simulink model "quad_new_leg_raibert_strategy_v2"  (R2022b)
settings: Solver=ode15s  StartTime=0.0  StopTime=400  RelTol=1e-3
InitFcn:
  | init_quad_new_leg_raibert_strategy_v2
values from neighbouring files (symbols this model uses):
  body = 'obstacle'+string(i)    [GUIWithNavigation.m]    (also in RunModel.m)
  floorl = 20    [EnvironmentData.mat]    (also in GUIWithNavigation.m; Practice data.mat; RunModel.m)
  floorw = 20    [EnvironmentData.mat]    (also in GUIWithNavigation.m; Practice data.mat; RunModel.m)
  planner = plannerRRTStar(ss,stateValidator)    [GUIWithNavigation.m]    (also in RunModel.m)
  startx = 3    [EnvironmentData.mat]    (also in Practice data.mat = 2)
  starty = 3    [EnvironmentData.mat]    (also in Practice data.mat = 2)
  tar1Len = 10    [EnvironmentData.mat]    (also in GUIWithNavigation.m = length(target1); Practice data.mat = 13; RunModel.m = length(target1))
  target = [3 4.99844642156 6.95141646815 8.78790598722 9.67257563911 9.70990834754 10.5092252376 9.30187214417 9.05327436398 9.4 9.4 10.8486938703 ... (44 elements, 22x2)]    [EnvironmentData.mat]    (also in GUIWithNavigation.m = cat(1,target1,target2); Practice data.mat = [2 3.44057581018 5.07942513831 5.42542290116 7.21306818311 8; RunModel.m = cat(1,target1,target2))
undefined symbols (not defined in the file or in its folder): closeFingers, ctrl, Extr_Data_LinkEndHole, grabObjectAngles, grabObjectAngles2, ground, holdFingers, l1, l2, m1, m2, openFingers, readyAngles, X, Y, Z
libraries: sm_lib x277, nesl_utility x98, slpidlib x31, simulink x5, Contact_Forces_Lib x4, Parts_Lib x4, sharedtransform x2
(part 1 of 11)
settings Model: Creator=biorobotics  LastModifiedBy=Harry
settings SolverCC: AlgebraicLoopSolver=TrustRegion
settings DataIOCC: ReturnWorkspaceOutputs=off
settings DebuggingCC: UnconnectedInputMsg=warning  UnconnectedOutputMsg=warning  UnconnectedLineMsg=warning  SFMachineParentedDataDiag=warning  ArithmeticOperatorsInVariantConditions=warning
settings ModelReferenceCC: EnableRefExpFcnMdlSchedulingChecks=on
settings SFSimCC: SimUseLocalCustomCode=off  CustomCodeUndefinedFunction=UseInterfaceOnly
settings RTWCC: RTWUseLocalCustomCode=off
settings DiagnosticsConfigSet: SimMechanicsRigidlyBoundBlock=none

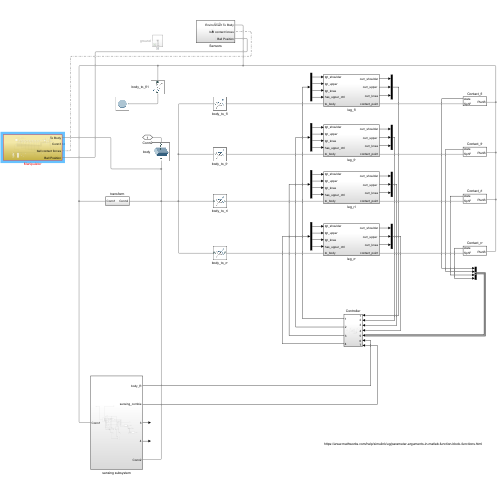
[thumbnail: Simulink's stored preview of the top-level diagram]
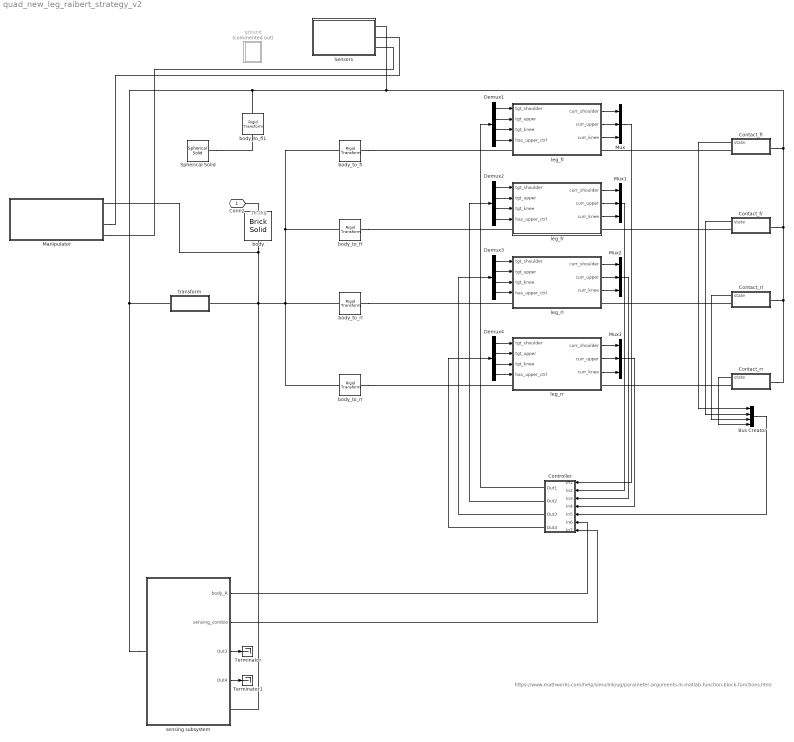
== system quad_new_leg_raibert_strategy_v2 ==
  note: 16.2kg
  note: https://www.mathworks.com/help/simulink/ug/parameter-arguments-in-matlab-function-block-functions.html
  Bus Creator : BusCreator  Inputs=4
  Contact_fl : Subsystem
  Contact_fr : Subsystem
  Contact_rl : Subsystem
  Contact_rr : Subsystem
  Controller : Subsystem
  Demux{1..4} (4 alike) : Demux
  Manipulator : Subsystem
  Mux{,1..3} (4 alike) : Mux  Inputs=3
  Sensors : Subsystem
  Spherical Solid : sm_lib/Body Elements/Spherical Solid  GraphicAmbientColor=[0.15 0.15 0.15 1.0]  BasedOnType=Density  CenterOfMass=[0 0 0]  CenterOfMassUnits=m  GraphicDiffuseColor=[0.4 0.2 0.0]  Density=1000  DensityUnits=kg/m^3  DoExposeReferenceFrame=on  GraphicEmissiveColor=[0.0 0.0 0.0 1.0]  ExportEntireGeometry=off  SerializedExposedGeometries=<ExposedGeometries/>  SerializedFrames=<Frames/>  MarkerShape=Sphere  MarkerSize=10  GraphicType=FromGeometry  InertiaType=CalculateFromGeometry  Mass=1  MassUnits=kg  MomentsOfInertia=[1 1 1]  MomentsOfInertiaUnits=kg*m^2  GraphicOpacity=1.0  ProductsOfInertia=[0 0 0]  ProductsOfInertiaUnits=kg*m^2  GraphicShininess=75  GraphicSpecularColor=[0.5 0.5 0.5 1.0]  SphereRadius=0.1  SphereRadiusUnits=m  GraphicVisPropType=SimpleVisualProperties
  Terminator : Terminator
  Terminator1 : Terminator
  body : sm_lib/Body Elements/Brick Solid  GraphicAmbientColor=[0.15 0.15 0.15 1.0]  BasedOnType=Density  BrickDimensions=[body.x_length body.y_length body.z_length]  BrickDimensionUnits=m  CenterOfMass=[0 0 0]  CenterOfMassUnits=m  GraphicDiffuseColor=[164 184 200]/255  Density=600  DensityUnits=kg/(m^3)  DoExposeReferenceFrame=on  GraphicEmissiveColor=[0.0 0.0 0.0 1.0]  ExportEntireGeometry=off  SerializedFrames=<Frames><Frame><Id>Frame2</Id><Value><Name>force</Name><Origin><Source>CenterOfMassFrame</Source><FeatureName></FeatureName></Origin><PrimaryAxis><DefinedDirection>+Z</DefinedDirection><Source>ReferenceFrame</Source><SourceDirection>+Z</SourceDirection><FeatureName></FeatureName></PrimaryAxis><SecondaryAxis><DefinedDirection>+X</DefinedDirection><Source>ReferenceFrame</Source><SourceDirection>+X</SourceDirection><FeatureName></FeatureName></SecondaryAxis></Value></Frame></Frames>  MarkerShape=Sphere  MarkerSize=10  GraphicType=FromGeometry  InertiaType=CalculateFromGeometry  Mass=8.6  MassUnits=kg  MomentsOfInertia=[1 1 1]  MomentsOfInertiaUnits=kg*m^2  GraphicOpacity=1.0  ProductsOfInertia=[0 0 0]  ProductsOfInertiaUnits=kg*m^2  GraphicShininess=75  GraphicSpecularColor=[0.5 0.5 0.5 1.0]  GraphicVisPropType=SimpleVisualProperties
  body_to_fl : sm_lib/Frames and Transforms/Rigid Transform  TranslationMethod=Cartesian  TranslationStandardOffset=0  TranslationLengthUnit=m  TranslationStandardAxis=+Z  TranslationCartesianOffset=[body.shoulder_distance body.y_length/2+body.shoulder_size/2 0]  TranslationROffset=0  TranslationROffsetUnits=m  TranslationZOffset=0  TranslationZOffsetUnits=m  TranslationThetaOffset=0  TranslationThetaOffsetUnits=deg  RotationMethod=AlignedAxes  RotationAngleUnits=deg  RotationStandardAxis=+Z  RotationAngle=0.0  RotationArbitraryAxis=[0 0 1]  FollAlignAxisA=+Z  BaseAlignAxisA=+X  FollAlignAxisB=+X  BaseAlignAxisB=-Z  RotationSequenceAxes=FollowerAxes  RotationSequence=XYX  RotationSequenceAngles=[0 0 0]  RotationSequenceAnglesUnits=deg  RotationMatrix=[1 0 0; 0 1 0; 0 0 1]  Quaternion=[1 0 0 0]
  body_to_fl1 : sm_lib/Frames and Transforms/Rigid Transform  TranslationMethod=Cartesian  TranslationStandardOffset=0  TranslationLengthUnit=m  TranslationStandardAxis=+Z  TranslationCartesianOffset=[1 -1 0]  TranslationROffset=0  TranslationROffsetUnits=m  TranslationZOffset=0  TranslationZOffsetUnits=m  TranslationThetaOffset=0  TranslationThetaOffsetUnits=deg  RotationMethod=None  RotationAngleUnits=deg  RotationStandardAxis=+Z  RotationAngle=0.0  RotationArbitraryAxis=[0 0 1]  FollAlignAxisA=+Z  BaseAlignAxisA=+X  FollAlignAxisB=+X  BaseAlignAxisB=-Z  RotationSequenceAxes=FollowerAxes  RotationSequence=XYX  RotationSequenceAngles=[0 0 0]  RotationSequenceAnglesUnits=deg  RotationMatrix=[1 0 0; 0 1 0; 0 0 1]  Quaternion=[1 0 0 0]
  body_to_fr : sm_lib/Frames and Transforms/Rigid Transform  TranslationMethod=Cartesian  TranslationStandardOffset=0  TranslationLengthUnit=m  TranslationStandardAxis=+Z  TranslationCartesianOffset=[body.shoulder_distance -body.y_length/2-body.shoulder_size/2 0]  TranslationROffset=0  TranslationROffsetUnits=m  TranslationZOffset=0  TranslationZOffsetUnits=m  TranslationThetaOffset=0  TranslationThetaOffsetUnits=deg  RotationMethod=AlignedAxes  RotationAngleUnits=deg  RotationStandardAxis=+Z  RotationAngle=0.0  RotationArbitraryAxis=[0 0 1]  FollAlignAxisA=+Z  BaseAlignAxisA=+X  FollAlignAxisB=+X  BaseAlignAxisB=-Z  RotationSequenceAxes=FollowerAxes  RotationSequence=XYX  RotationSequenceAngles=[0 0 0]  RotationSequenceAnglesUnits=deg  RotationMatrix=[1 0 0; 0 1 0; 0 0 1]  Quaternion=[1 0 0 0]
  body_to_rl : sm_lib/Frames and Transforms/Rigid Transform  TranslationMethod=Cartesian  TranslationStandardOffset=0  TranslationLengthUnit=m  TranslationStandardAxis=+Z  TranslationCartesianOffset=[-body.shoulder_distance body.y_length/2+body.shoulder_size/2 0]  TranslationROffset=0  TranslationROffsetUnits=m  TranslationZOffset=0  TranslationZOffsetUnits=m  TranslationThetaOffset=0  TranslationThetaOffsetUnits=deg  RotationMethod=AlignedAxes  RotationAngleUnits=deg  RotationStandardAxis=+Z  RotationAngle=0.0  RotationArbitraryAxis=[0 0 1]  FollAlignAxisA=+Z  BaseAlignAxisA=+X  FollAlignAxisB=+X  BaseAlignAxisB=-Z  RotationSequenceAxes=FollowerAxes  RotationSequence=XYX  RotationSequenceAngles=[0 0 0]  RotationSequenceAnglesUnits=deg  RotationMatrix=[1 0 0; 0 1 0; 0 0 1]  Quaternion=[1 0 0 0]
  body_to_rr : sm_lib/Frames and Transforms/Rigid Transform  TranslationMethod=Cartesian  TranslationStandardOffset=0  TranslationLengthUnit=m  TranslationStandardAxis=+Z  TranslationCartesianOffset=[-body.shoulder_distance -body.y_length/2-body.shoulder_size/2 0]  TranslationROffset=0  TranslationROffsetUnits=m  TranslationZOffset=0  TranslationZOffsetUnits=m  TranslationThetaOffset=0  TranslationThetaOffsetUnits=deg  RotationMethod=AlignedAxes  RotationAngleUnits=deg  RotationStandardAxis=+Z  RotationAngle=0.0  RotationArbitraryAxis=[0 0 1]  FollAlignAxisA=+Z  BaseAlignAxisA=+X  FollAlignAxisB=+X  BaseAlignAxisB=-Z  RotationSequenceAxes=FollowerAxes  RotationSequence=XYX  RotationSequenceAngles=[0 0 0]  RotationSequenceAnglesUnits=deg  RotationMatrix=[1 0 0; 0 1 0; 0 0 1]  Quaternion=[1 0 0 0]
  ground : Subsystem  Commented=on
  leg_fl : Subsystem
  leg_fr : Subsystem
  leg_rl : Subsystem
  leg_rr : Subsystem
  "sensing subsystem " : Subsystem
  transform : Subsystem
  Conn2 : PMIOPort  Side=Left
  wires:
  Demux1/1 -> leg_fl/1(tgt_shoulder)
  Mux/1 -> Controller/1(In1)
  Demux3/1 -> leg_rl/1(tgt_shoulder)
  leg_fr/1(curr_shoulder) -> Mux1/1
  leg_fl/1(curr_shoulder) -> Mux/1
  "sensing subsystem "/1(body_R) -> Controller/6(In6)
  Demux2/3 -> leg_fr/3(tgt_knee)
  leg_fr/3(curr_knee) -> Mux1/3
  Bus Creator/1 -> Controller/5(In5)
  leg_rr/3(curr_knee) -> Mux3/3
  "sensing subsystem "/4(Out4) -> Terminator1/1
  leg_fr/2("curr_upper ") -> Mux1/2
  Mux1/1 -> Controller/2(In2)
  leg_rl/3(curr_knee) -> Mux2/3
  leg_fl/2("curr_upper ") -> Mux/2
  Contact_fr/1(state) -> Bus Creator/2
  leg_fl/3(curr_knee) -> Mux/3
  leg_rl/1(curr_shoulder) -> Mux2/1
  Contact_rl/1(state) -> Bus Creator/3
  leg_rl/2("curr_upper ") -> Mux2/2
  Demux4/2 -> leg_rr/2(tgt_upper)
  leg_rr/1(curr_shoulder) -> Mux3/1
  Controller/4(Out4) -> Demux4/1
  Mux3/1 -> Controller/4(In4)
  leg_rr/2("curr_upper ") -> Mux3/2
  Demux4/3 -> leg_rr/3(tgt_knee)
  Mux2/1 -> Controller/3(In3)
  Demux4/4 -> leg_rr/4(has_upper_ctrl)
  Controller/2(Out2) -> Demux2/1
  "sensing subsystem "/2(sensing_combie) -> Controller/7(In7)
  Demux2/4 -> leg_fr/4(has_upper_ctrl)
  "sensing subsystem "/3(Out3) -> Terminator/1
  Demux1/2 -> leg_fl/2(tgt_upper)
  Demux3/2 -> leg_rl/2(tgt_upper)
  Demux1/3 -> leg_fl/3(tgt_knee)
  Demux2/2 -> leg_fr/2(tgt_upper)
  Demux4/1 -> leg_rr/1(tgt_shoulder)
  Demux3/3 -> leg_rl/3(tgt_knee)
  Contact_fl/1(state) -> Bus Creator/1
  Controller/1(Out1) -> Demux1/1
  Demux1/4 -> leg_fl/4(has_upper_ctrl)
  Controller/3(Out3) -> Demux3/1
  Demux2/1 -> leg_fr/1(tgt_shoulder)
  Contact_rr/1(state) -> Bus Creator/4
  Demux3/4 -> leg_rl/4(has_upper_ctrl)
  connections:
  "sensing subsystem "/RConn1 -- Manipulator/RConn1 -- body/RConn1 -- transform/LConn1 -- body_to_rl/LConn1 -- body_to_rr/LConn1 -- body_to_fl/LConn1 -- body_to_fr/LConn1
  body_to_rl/RConn1 -- leg_rl/LConn1
  body_to_fl/RConn1 -- leg_fl/LConn1
  body/LConn1 -- Conn2/RConn1
  Contact_fl/RConn1 -- leg_fl/RConn1
  body_to_fr/RConn1 -- leg_fr/LConn1
  Contact_rl/RConn1 -- leg_rl/RConn1
  body_to_rr/RConn1 -- leg_rr/LConn1
  Contact_fr/RConn1 -- leg_fr/RConn1
  Spherical Solid/RConn1 -- body_to_fl1/RConn1
  Contact_rr/RConn1 -- leg_rr/RConn1
  "sensing subsystem "/LConn1 -- Sensors/RConn1 -- Contact_fr/LConn1 -- Contact_rr/LConn1 -- Contact_rl/LConn1 -- Contact_fl/LConn1 -- body_to_fl1/LConn1 -- transform/RConn1
  Manipulator/RConn3 -- Sensors/RConn2
  Manipulator/RConn4 -- Sensors/RConn3

== system quad_new_leg_raibert_strategy_v2/Contact_fl ==
  note: state 4 166.31ms
  note: 这是一个蛋疼的处理，因为地面现在厚度是0.4，为了和碰撞的block要求匹配，所以碰撞是相对于这个地面的中心来算的。而检测高度的时候就要把这个厚度减掉
      | 但是Transform sensor要检测的是球和地面的高度差
  Bus Selector : BusSelector  OutputSignals=Normal Force,Frame Sep,Friction Force
  Compare To Constant : simulink/Logic and Bit Operations/Compare To Constant  relop=<=  const=planner.touch_down_height  OutDataTypeStr=uint8
  PSConv4 : nesl_utility/PS-Simulink Converter  PhysicalDomain=network_engine_domain  SubClassName=ps_output  LeftPortType=input  RightPortType=output  PseudoPeriodic=off  Frequencies=[]  VectorFormat=1-D array  Unit=1  AffineConversion=off
  Sphere to Plane Force1 : Contact_Forces_Lib/3D/Sphere to Plane Force  sphere_rad=body.foot_radius  plane_lenx=40  plane_leny=40  plane_depth=0  force_law=Linear  k_contact=ground.stiff  b_contact=ground.damp  pen_full_damp_F=1e-4  pen_exponent=1  custom_param_1=1  custom_param_2=1  friction_law=Stick-Slip Continuous  mu_kinetic=0.7  mu_static=0.7  v_thr=0.001  vis_on=off  vis_opc_en=0  vis_len_plaBz=0.005  vis_clr=[0.9 0.2 0.2]  vis_opc=0.7
  State Scope : Scope
  Terminator : Terminator
  Transform Sensor : sm_lib/Frames and Transforms/Transform Sensor  MeasurementFrame=World  SenseAngle=off  SenseAxis=off  SenseQ=off  SenseR=off  SenseRotationSequence=off  RotationSequence=XYX  SenseOmegaX=off  SenseOmegaY=off  SenseOmegaZ=off  SenseQDot=off  SenseRDot=off  SenseAlphaX=off  SenseAlphaY=off  SenseAlphaZ=off  SenseQDDot=off  SenseRDDot=off  SenseX=off  SenseY=off  SenseZ=on  SenseRad=off  SenseAzim=off  SenseDist=off  SenseInc=off  SenseXDot=off  SenseYDot=off  SenseZDot=off  SenseRadDot=off  SenseAzimDot=off  SenseDistDot=off  SenseIncDot=off  SenseXDDot=off  SenseYDDot=off  SenseZDDot=off  SenseRadDDot=off  SenseAzimDDot=off  SenseDistDDot=off  SenseIncDDot=off
  ZScope : Scope
  force : Scope  NumInputPorts=2
  PlanB : PMIOPort  Side=Left
  SphF : PMIOPort  Port=2  Side=Right
  state : Outport  VectorParamsAs1DForOutWhenUnconnected=off
  wires:
  Sphere to Plane Force1/1 -> Bus Selector/1
  Bus Selector/1 -> force/1  "<Normal Force>"
  PSConv4/1 -> Compare To Constant/1, ZScope/1
  Compare To Constant/1 -> state/1, State Scope/1
  Bus Selector/3 -> force/2  "<Friction Force>"
  Bus Selector/2 -> Terminator/1  "<Frame Sep>"
  connections:
  Sphere to Plane Force1/LConn1 -- Transform Sensor/RConn1 -- SphF/RConn1
  Sphere to Plane Force1/RConn1 -- Transform Sensor/LConn1 -- PlanB/RConn1
  PSConv4/LConn1 -- Transform Sensor/RConn2

== system quad_new_leg_raibert_strategy_v2/Contact_fr ==
  note: state 4 166.31ms
  note: 这是一个蛋疼的处理，因为地面现在厚度是0.4，为了和碰撞的block要求匹配，所以碰撞是相对于这个地面的中心来算的。而检测高度的时候就要把这个厚度减掉
      | 但是Transform sensor要检测的是球和地面的高度差
  Bus Selector : BusSelector  OutputSignals=Normal Force,Frame Sep,Friction Force
  Compare To Constant : simulink/Logic and Bit Operations/Compare To Constant  relop=<=  const=planner.touch_down_height  OutDataTypeStr=uint8
  PSConv4 : nesl_utility/PS-Simulink Converter  PhysicalDomain=network_engine_domain  SubClassName=ps_output  LeftPortType=input  RightPortType=output  PseudoPeriodic=off  Frequencies=[]  VectorFormat=1-D array  Unit=1  AffineConversion=off
  Sphere to Plane Force1 : Contact_Forces_Lib/3D/Sphere to Plane Force  sphere_rad=body.foot_radius  plane_lenx=40  plane_leny=40  plane_depth=0  force_law=Linear  k_contact=ground.stiff  b_contact=ground.damp  pen_full_damp_F=1e-4  pen_exponent=1  custom_param_1=1  custom_param_2=1  friction_law=Stick-Slip Continuous  mu_kinetic=0.7  mu_static=0.7  v_thr=0.001  vis_on=off  vis_opc_en=0  vis_len_plaBz=0.005  vis_clr=[0.9 0.2 0.2]  vis_opc=0.7
  State Scope : Scope
  Terminator : Terminator
  Transform Sensor : sm_lib/Frames and Transforms/Transform Sensor  MeasurementFrame=World  SenseAngle=off  SenseAxis=off  SenseQ=off  SenseR=off  SenseRotationSequence=off  RotationSequence=XYX  SenseOmegaX=off  SenseOmegaY=off  SenseOmegaZ=off  SenseQDot=off  SenseRDot=off  SenseAlphaX=off  SenseAlphaY=off  SenseAlphaZ=off  SenseQDDot=off  SenseRDDot=off  SenseX=off  SenseY=off  SenseZ=on  SenseRad=off  SenseAzim=off  SenseDist=off  SenseInc=off  SenseXDot=off  SenseYDot=off  SenseZDot=off  SenseRadDot=off  SenseAzimDot=off  SenseDistDot=off  SenseIncDot=off  SenseXDDot=off  SenseYDDot=off  SenseZDDot=off  SenseRadDDot=off  SenseAzimDDot=off  SenseDistDDot=off  SenseIncDDot=off
  ZScope : Scope
  force : Scope  NumInputPorts=2
  PlanB : PMIOPort  Side=Left
  SphF : PMIOPort  Port=2  Side=Right
  state : Outport  VectorParamsAs1DForOutWhenUnconnected=off
  wires:
  Sphere to Plane Force1/1 -> Bus Selector/1
  Bus Selector/1 -> force/1  "<Normal Force>"
  PSConv4/1 -> Compare To Constant/1, ZScope/1
  Compare To Constant/1 -> state/1, State Scope/1
  Bus Selector/3 -> force/2  "<Friction Force>"
  Bus Selector/2 -> Terminator/1  "<Frame Sep>"
  connections:
  Sphere to Plane Force1/LConn1 -- Transform Sensor/RConn1 -- SphF/RConn1
  Sphere to Plane Force1/RConn1 -- Transform Sensor/LConn1 -- PlanB/RConn1
  PSConv4/LConn1 -- Transform Sensor/RConn2

== system quad_new_leg_raibert_strategy_v2/Contact_rl ==
  note: 这是一个蛋疼的处理，因为地面现在厚度是0.4，为了和碰撞的block要求匹配，所以碰撞是相对于这个地面的中心来算的。而检测高度的时候就要把这个厚度减掉
      | 但是Transform sensor要检测的是球和地面的高度差
  Bus Selector : BusSelector  OutputSignals=Normal Force,Frame Sep,Friction Force
  Compare To Constant : simulink/Logic and Bit Operations/Compare To Constant  relop=<=  const=planner.touch_down_height  OutDataTypeStr=uint8
  PSConv4 : nesl_utility/PS-Simulink Converter  PhysicalDomain=network_engine_domain  SubClassName=ps_output  LeftPortType=input  RightPortType=output  PseudoPeriodic=off  Frequencies=[]  VectorFormat=1-D array  Unit=1  AffineConversion=off
  Sphere to Plane Force1 : Contact_Forces_Lib/3D/Sphere to Plane Force  sphere_rad=body.foot_radius  plane_lenx=40  plane_leny=40  plane_depth=0  force_law=Linear  k_contact=ground.stiff  b_contact=ground.damp  pen_full_damp_F=1e-4  pen_exponent=1  custom_param_1=1  custom_param_2=1  friction_law=Stick-Slip Continuous  mu_kinetic=0.7  mu_static=0.7  v_thr=0.001  vis_on=off  vis_opc_en=0  vis_len_plaBz=0.005  vis_clr=[0.9 0.2 0.2]  vis_opc=0.7
  State Scope : Scope
  Terminator : Terminator
  Transform Sensor : sm_lib/Frames and Transforms/Transform Sensor  MeasurementFrame=World  SenseAngle=off  SenseAxis=off  SenseQ=off  SenseR=off  SenseRotationSequence=off  RotationSequence=XYX  SenseOmegaX=off  SenseOmegaY=off  SenseOmegaZ=off  SenseQDot=off  SenseRDot=off  SenseAlphaX=off  SenseAlphaY=off  SenseAlphaZ=off  SenseQDDot=off  SenseRDDot=off  SenseX=off  SenseY=off  SenseZ=on  SenseRad=off  SenseAzim=off  SenseDist=off  SenseInc=off  SenseXDot=off  SenseYDot=off  SenseZDot=off  SenseRadDot=off  SenseAzimDot=off  SenseDistDot=off  SenseIncDot=off  SenseXDDot=off  SenseYDDot=off  SenseZDDot=off  SenseRadDDot=off  SenseAzimDDot=off  SenseDistDDot=off  SenseIncDDot=off
  ZScope : Scope
  force : Scope  NumInputPorts=2
  PlanB : PMIOPort  Side=Left
  SphF : PMIOPort  Port=2  Side=Right
  state : Outport  VectorParamsAs1DForOutWhenUnconnected=off
  wires:
  Sphere to Plane Force1/1 -> Bus Selector/1
  Bus Selector/1 -> force/1  "<Normal Force>"
  PSConv4/1 -> Compare To Constant/1, ZScope/1
  Compare To Constant/1 -> state/1, State Scope/1
  Bus Selector/3 -> force/2  "<Friction Force>"
  Bus Selector/2 -> Terminator/1  "<Frame Sep>"
  connections:
  Sphere to Plane Force1/LConn1 -- Transform Sensor/RConn1 -- SphF/RConn1
  Sphere to Plane Force1/RConn1 -- Transform Sensor/LConn1 -- PlanB/RConn1
  PSConv4/LConn1 -- Transform Sensor/RConn2

== system quad_new_leg_raibert_strategy_v2/Contact_rr ==
  note: state 4 166.31ms
  note: 这是一个蛋疼的处理，因为地面现在厚度是0.4，为了和碰撞的block要求匹配，所以碰撞是相对于这个地面的中心来算的。而检测高度的时候就要把这个厚度减掉
      | 但是Transform sensor要检测的是球和地面的高度差
  Bus Selector : BusSelector  OutputSignals=Normal Force,Frame Sep,Friction Force
  Compare To Constant : simulink/Logic and Bit Operations/Compare To Constant  relop=<=  const=planner.touch_down_height  OutDataTypeStr=uint8
  PSConv4 : nesl_utility/PS-Simulink Converter  PhysicalDomain=network_engine_domain  SubClassName=ps_output  LeftPortType=input  RightPortType=output  PseudoPeriodic=off  Frequencies=[]  VectorFormat=1-D array  Unit=1  AffineConversion=off
  Sphere to Plane Force1 : Contact_Forces_Lib/3D/Sphere to Plane Force  sphere_rad=body.foot_radius  plane_lenx=40  plane_leny=40  plane_depth=0  force_law=Linear  k_contact=ground.stiff  b_contact=ground.damp  pen_full_damp_F=1e-4  pen_exponent=1  custom_param_1=1  custom_param_2=1  friction_law=Stick-Slip Continuous  mu_kinetic=0.7  mu_static=0.7  v_thr=0.001  vis_on=off  vis_opc_en=0  vis_len_plaBz=0.005  vis_clr=[0.9 0.2 0.2]  vis_opc=0.7
  State Scope : Scope
  Terminator : Terminator
  Transform Sensor : sm_lib/Frames and Transforms/Transform Sensor  MeasurementFrame=World  SenseAngle=off  SenseAxis=off  SenseQ=off  SenseR=off  SenseRotationSequence=off  RotationSequence=XYX  SenseOmegaX=off  SenseOmegaY=off  SenseOmegaZ=off  SenseQDot=off  SenseRDot=off  SenseAlphaX=off  SenseAlphaY=off  SenseAlphaZ=off  SenseQDDot=off  SenseRDDot=off  SenseX=off  SenseY=off  SenseZ=on  SenseRad=off  SenseAzim=off  SenseDist=off  SenseInc=off  SenseXDot=off  SenseYDot=off  SenseZDot=off  SenseRadDot=off  SenseAzimDot=off  SenseDistDot=off  SenseIncDot=off  SenseXDDot=off  SenseYDDot=off  SenseZDDot=off  SenseRadDDot=off  SenseAzimDDot=off  SenseDistDDot=off  SenseIncDDot=off
  ZScope : Scope
  force : Scope  NumInputPorts=2
  PlanB : PMIOPort  Side=Left
  SphF : PMIOPort  Port=2  Side=Right
  state : Outport  VectorParamsAs1DForOutWhenUnconnected=off
  wires:
  Sphere to Plane Force1/1 -> Bus Selector/1
  Bus Selector/1 -> force/1  "<Normal Force>"
  PSConv4/1 -> Compare To Constant/1, ZScope/1
  Compare To Constant/1 -> state/1, State Scope/1
  Bus Selector/3 -> force/2  "<Friction Force>"
  Bus Selector/2 -> Terminator/1  "<Frame Sep>"
  connections:
  Sphere to Plane Force1/LConn1 -- Transform Sensor/RConn1 -- SphF/RConn1
  Sphere to Plane Force1/RConn1 -- Transform Sensor/LConn1 -- PlanB/RConn1
  PSConv4/LConn1 -- Transform Sensor/RConn2

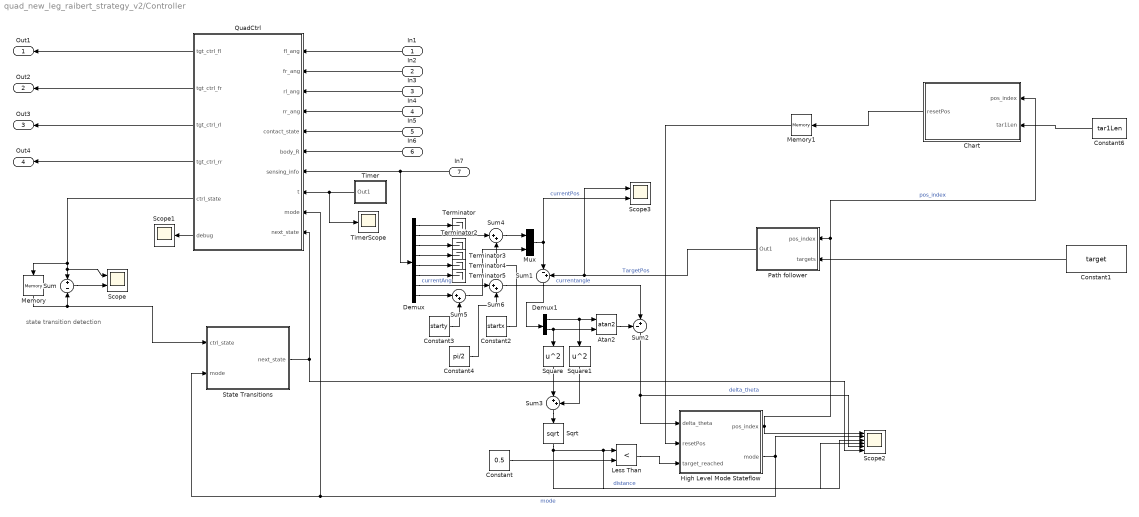
== system quad_new_leg_raibert_strategy_v2/Controller ==
  note: state transition detection
  In1 : Inport
  In2 : Inport  Port=2
  In3 : Inport  Port=3
  In4 : Inport  Port=4
  In5 : Inport  Port=5
  In6 : Inport  Port=6
  In7 : Inport  Port=7
  Atan2 : Trigonometry  Operator=atan2
  Chart : Stateflow chart  TreatAsAtomicUnit=on
  Constant : Constant  Value=0.5
  Constant1 : Constant  Value=target
  Constant2 : Constant  Value=startx
  Constant3 : Constant  Value=starty
  Constant4 : Constant  Value=pi/2
  Constant6 : Constant  Value=tar1Len
  Demux : Demux  Outputs=8
  Demux1 : Demux  Outputs=2
  High Level Mode Stateflow : Stateflow chart  TreatAsAtomicUnit=on
      settings: PortSchema="{\"entries\":[{\"content\":{\"sides\":[{\"content\":{\"connectorIds\":[\"In2\",\"In3\",\"In1\"]},\"type\":\"ConnectorPlacement.EquallySpacedRectSide\",\"uuid\":\"54635eaa-af22-4c07-946c-8b3764ca4079\"},{\"content\":{\"connectorIds\":[\"Out1\",\"Out2\"],\"side\":\"RIGHT\"},\"type\":\"ConnectorPlacement.EquallySpacedRectSide\",\"uuid\":\"b8ca9e50-c21e-481d-aebe-d3447dd5b6ec\"},{\"content\":{\"connectorIds\":[],\"side\":\"TOP\"},\"type\":\"ConnectorPlacement.EquallySpacedRectSide\",\"uuid\":\"aa364018-0c1f-4137-8fa7-722b902e07a1\"}]},\"type\":\"ConnectorPlacement.EquallySpacedConnector\",\"uuid\":\"b87c06e7-bef4-4368-b066-66035be64295\"}],\"packageUris\":[\"http://schema.mathworks.com/mf0/Connector/R2020b\"],\"version\":\"1.0\"}"
  Less Than : RelationalOperator  Operator=<  OutDataTypeStr=boolean  RndMeth=Simplest  InputSameDT=off
  Memory : Memory
  Memory1 : Memory
  Mux : Mux  Inputs=2
  Path follower : Subsystem  TreatAsAtomicUnit=on
  QuadCtrl : MATLAB Function  TreatAsAtomicUnit=on  SystemSampleTime=0.0025
  Scope : Scope  NumInputPorts=2
  Scope1 : Scope
  Scope2 : Scope  NumInputPorts=6
  Scope3 : Scope  NumInputPorts=2
  Sqrt : Sqrt
  Square : Math  Operator=square
  Square1 : Math  Operator=square
  State Transitions : Stateflow chart  TreatAsAtomicUnit=on
  Sum : Sum  Inputs=+-
  Sum1 : Sum  Inputs=|-+
  Sum2 : Sum  Inputs=-+|
  Sum{3..6} (4 alike) : Sum  Inputs=|++
  Terminator{,2..5} (5 alike) : Terminator
  Timer : Subsystem
  TimerScope : Scope
  Out1 : Outport  VectorParamsAs1DForOutWhenUnconnected=off
  Out2 : Outport  Port=2  VectorParamsAs1DForOutWhenUnconnected=off
  Out3 : Outport  Port=3  VectorParamsAs1DForOutWhenUnconnected=off
  Out4 : Outport  Port=4  VectorParamsAs1DForOutWhenUnconnected=off
  wires:
  In7/1 -> Demux/1, QuadCtrl/7(sensing_info)
  In4/1 -> QuadCtrl/4(rr_ang)
  Timer/1(Out1) -> TimerScope/1, QuadCtrl/8(t)
  In3/1 -> QuadCtrl/3(rl_ang)
  In5/1 -> QuadCtrl/5(contact_state)
  In1/1 -> QuadCtrl/1(fl_ang)
  QuadCtrl/3(tgt_ctrl_rl) -> Out3/1
  In6/1 -> QuadCtrl/6(body_R)
  QuadCtrl/2(tgt_ctrl_fr) -> Out2/1
  In2/1 -> QuadCtrl/2(fr_ang)
  QuadCtrl/4(tgt_ctrl_rr) -> Out4/1
  QuadCtrl/1(tgt_ctrl_fl) -> Out1/1
  QuadCtrl/5(ctrl_state) -> Scope/1, Sum/1, Memory/1
  Memory/1 -> State Transitions/1(ctrl_state), Sum/2
  Sum/1 -> Scope/2
  QuadCtrl/6(debug) -> Scope1/1
  Less Than/1 -> High Level Mode Stateflow/1(target_reached)
  Sum2/1 -> Scope2/5, High Level Mode Stateflow/2(delta_theta)  "delta_theta"
  High Level Mode Stateflow/1(pos_index) -> Chart/1(pos_index), Path follower/1(pos_index), Scope2/1  "pos_index"
  High Level Mode Stateflow/2(mode) -> QuadCtrl/9(mode), State Transitions/2(mode), Scope2/2  "mode"
  Demux/1 -> Terminator/1
  Demux/3 -> Terminator2/1
  Demux/4 -> Terminator3/1
  Demux/5 -> Terminator4/1
  Demux/6 -> Terminator5/1
  Mux/1 -> Scope3/2, Sum1/1  "currentPos"
  Sum1/1 -> Demux1/1
  Demux1/1 -> Square1/1, Atan2/1
  Demux1/2 -> Atan2/2, Square/1
  Atan2/1 -> Sum2/1
  Sum3/1 -> Sqrt/1
  Square1/1 -> Sum3/2
  Square/1 -> Sum3/1
  Sqrt/1 -> Scope2/3, Scope2/4, Less Than/1  "distance"
  Constant/1 -> Less Than/2
  State Transitions/1(next_state) -> Scope2/6, QuadCtrl/10(next_state)
  Path follower/1(Out1) -> Scope3/1, Sum1/2  "TargetPos"
  Demux/2 -> Sum4/1
  Demux/8 -> Sum5/1
  Constant2/1 -> Sum4/2
  Constant3/1 -> Sum5/2
  Sum4/1 -> Mux/1
  Sum5/1 -> Mux/2
  Constant4/1 -> Sum6/2
  Demux/7 -> Sum6/1  "currentAng"
  Sum6/1 -> Sum2/2  "currentangle"
  Constant6/1 -> Chart/2(tar1Len)
  Chart/1(resetPos) -> Memory1/1
  Memory1/1 -> High Level Mode Stateflow/3(resetPos)
  Constant1/1 -> Path follower/2(targets)
